simulink model "ORC_test_simu_unregSCIG"  (R2018a)
settings: Solver=FixedStepAuto  StartTime=0.0  StopTime=10  FixedStep=.1  RelTol=1e-4
values from neighbouring files (symbols this model uses):
  A_cond = 50    [Chena_ORC_test_simu_init.m]    (also in ORC_test_simu_init.m = 18.6)
  A_evap = 30    [Chena_ORC_test_simu_init.m]    (also in ORC_test_simu_init.m = 9.3)
  Cx = 620e-05    (= 0.0062)    [Chena_ORC_test_simu_init.m]    (also in ORC_test_simu_init.m = 0.000221048532072; SCIG_Admittance_Balance.m = 6.9e-05; SCIG_Energy_Balance_excitation.m = 1.35135135135; SCIG_Energy_Balance_excitation_sym.m = 5)
  eff_inverter = 0.93    [Chena_ORC_test_simu_init.m]    (also in ORC_test_simu_init.m)
  eff_pump = 0.78    [Chena_ORC_test_simu_init.m]    (also in ORC_Energy_Balance.m = 0.7; ORC_test.m = 0.7; ORC_test_brownfield.m = 0.7; ORC_test_greenfield.m = 0.7)
  eff_turbine = 0.8    [Chena_ORC_test_simu_init.m]    (also in ORC_test_simu_init.m = 0.78)
  f_rated = 60    [Chena_ORC_test_simu_init.m]    (also in ORC_test_simu_init.m; SCIG_Admittance_Balance.m; SCIG_Admittance_test.m; SCIG_Ouazenne.m)
  H_wf_init = 2.6e+05    (= 260000)    [Chena_ORC_test_simu_init.m]    (also in ORC_test_simu_init.m = 230000)
  Lr = 0.252/(2*pi*f_rated)/35    (= 1.9098593171e-05)    [Chena_ORC_test_simu_init.m]    (also in ORC_test_simu_init.m = 0.000132629119243)
  Ls = 0.423/(2*pi*f_rated)/35    (= 3.20583528228e-05)    [Chena_ORC_test_simu_init.m]    (also in ORC_test_simu_init.m = 0.000848826363157)
  m_dot_source = 33.39    [Chena_ORC_test_simu_init.m]    (also in ORC_Energy_Balance.m = 5.7714; ORC_test.m = 12; ORC_test_brownfield.m = 6; ORC_test_greenfield.m = 12)
  m_dot_wf_init = 12    [Chena_ORC_test_simu_init.m]    (also in ORC_test_simu_init.m = 3)
  m_dot_wf_max = 16    [Chena_ORC_test_simu_init.m]
  magCurveV = [98.1532063054068,98.8036071709152,99.4518999785459,100.098037520928,100.741973127402,101.383660677656,102.023054614968,102.660109959042,103.294782318460,103.927027902737,104.556803533993,105.184066658235,105.808775356268,106.430888354220,107.050365033694,107.667165441552,108.281250299330,108.892581012284,109.501119678081,110.106829095126,110.709672770539,111.309614927775,111.906620513896,112.5006 ...(+6146 chars)    [Chena_ORC_test_simu_init.m]    (also in ORC_test_simu_init.m = [21.5410077151772,22.1687511430959,22.7961934111159,23.42344)
  magCurveX = [0.663529769645709,0.663521969965503,0.663500208426959,0.663464444749194,0.663414643227627,0.663350772676200,0.663272806369214,0.663180721982808,0.663074501536138,0.662954131332260,0.662819601898778,0.662670907928276,0.662508048218555,0.662331025612717,0.662139846939116,0.661934522951205,0.661715068267290,0.661481501310239,0.661233844247137,0.660972122928937,0.660696366830103,0.660406608988283,0.6 ...(+6531 chars)    [Chena_ORC_test_simu_init.m]    (also in ORC_test_simu_init.m = [21.5410077151772,21.5637559851946,21.5850104594817,21.60498)
  p_atm = 101325    [Chena_ORC_test_simu_init.m]    (also in ORC_test_simu_init.m)
  pf_grid = 0.9    [Chena_ORC_test_simu_init.m]    (also in ORC_test_simu_init.m)
  poles = 2    [Chena_ORC_test_simu_init.m]    (also in Copy_of_SCIG_Energy_Balance_excitation.m = 4; SCIG_Admittance_Balance.m = 6; SCIG_Admittance_test.m = 6; SCIG_Ouazenne.m)
  Rr = 0.144/35    (= 0.00411428571429)    [Chena_ORC_test_simu_init.m]    (also in ORC_test_simu_init.m = 0.03)
  Rs = 0.148/35    (= 0.00422857142857)    [Chena_ORC_test_simu_init.m]    (also in ORC_test_simu_init.m = 0.018)
  Rx = 0    [Chena_ORC_test_simu_init.m]    (also in Copy_of_SCIG_Energy_Balance_excitation.m = 0.003; ORC_test_simu_init.m; SCIG_Admittance_Balance.m; SCIG_Admittance_test.m)
  Tin_sink = 277.59    [Chena_ORC_test_simu_init.m]    (also in ORC_test_simu_init.m = 278)
  Tin_source = 346.48    [Chena_ORC_test_simu_init.m]    (also in ORC_test_simu_init.m = 368)
  U_cond = 5000    [Chena_ORC_test_simu_init.m]    (also in ORC_test_simu_init.m = 1400)
  U_evap = 4500    [Chena_ORC_test_simu_init.m]    (also in ORC_test_simu_init.m = 1500)
  Vline_rated = 220    [Chena_ORC_test_simu_init.m]    (also in SCIG_Admittance_Balance.m = 6600; SCIG_Admittance_test.m = 6600; SCIG_Ouazenne.m; SCIG_Ouazenne_iterate.m)
  Xx = 1/(2*pi*f_rated*Cx)    (= 0.427835868527)    [Chena_ORC_test_simu_init.m]    (also in Copy_of_SCIG_Energy_Balance_excitation.m = 12; ORC_test_simu_init.m = 12; SCIG_Admittance_Balance.m = Xx(fvIDX); SCIG_Energy_Balance_excitation.m = 1./(Cx.*w_synch))
undefined symbols (not defined in the file or in its folder): handle_sink, handle_source, handle_wf, n_mech_init, n_mech_max, n_mech_min, sigbuilder_block
(part 1 of 4)
settings Model: Creator=njgreen3  LastModifiedBy=njgreen3
settings SolverCC: AlgebraicLoopSolver=LineSearch
settings DebuggingCC: ParameterOverflowMsg=warning

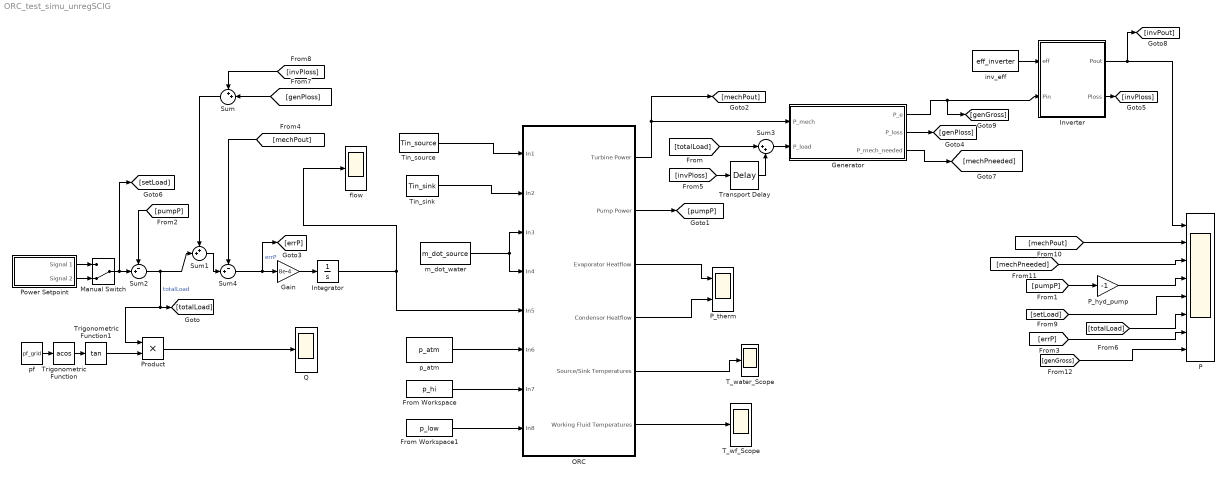
== system ORC_test_simu_unregSCIG ==
  From Workspace : FromWorkspace  VariableName=p_hi  SampleTime=0
  From Workspace1 : FromWorkspace  VariableName=p_low  SampleTime=0
  Gain : Gain  Gain=8e-4
  Generator : Subsystem
  Integrator : Integrator  InitialCondition=m_dot_wf_init  LimitOutput=on  UpperSaturationLimit=m_dot_wf_max  LowerSaturationLimit=0
  Inverter : MATLAB Function  TreatAsAtomicUnit=on
  Manual Switch : ManualSwitch  CurrentSetting=0
  ORC : Subsystem
  P : Scope  NumInputPorts=8
  P_hyd_pump : Gain  Gain=-1
  P_therm : Scope  NumInputPorts=2
  Power Setpoint : Subsystem  Tag=STV Subsys  LoadFcn=sigbuilder_block('load',[440.25 156.75 544.5 355.5 ]);  StartFcn=sigbuilder_block('start');  StopFcn=sigbuilder_block('stop');  ClipboardFcn=sigbuilder_block('clipboard');  mask(Sigbuilder block){tuvar=[0:10]}
      mask help: Simulink:masks:SigbuilderBlock_MD
      mask init:
      | if ~strcmp(get_param(bdroot(gcbh),'SimulationStatus'),'stopped') tuvar = sigbuilder_block('maskInit'); end
      settings: CopyFcn=sigbuilder_block('copy');  DeleteFcn=sigbuilder_block('delete');  ModelCloseFcn=sigbuilder_block('modelClose');  PreSaveFcn=sigbuilder_block('preSave');  PauseFcn=sigbuilder_block('pause');  ContinueFcn=sigbuilder_block('continue');  NameChangeFcn=sigbuilder_block('namechange');  OpenFcn=sigbuilder_block('open',[440.25 156.75 544.5 355.5 ]);  CloseFcn=sigbuilder_block('close');
      mask Display: plot(0, 0, 100, 100,[2, 2, 32, 32, 2], [68, 8, 8, 68, 68],[32, 2], [38, 38], [32, 19, 2],[53, 60, 44], [32, 17, 17, 2],[16, 16, 31, 31]);txt = getActiveGroup(gcbh);text(2, 100, txt,'verticalAlignment', 'top');
  Product : Product
  Q : Scope
  Sum : Sum  Inputs=++|
  Sum1 : Sum  Inputs=++|
  Sum2 : Sum  Inputs=-+|
  Sum3 : Sum  Inputs=|++
  Sum4 : Sum  Inputs=-+|
  T_water_Scope : Scope
  T_wf_Scope : Scope
  Tin_sink : Constant  Value=Tin_sink
  Tin_source : Constant  Value=Tin_source
  Transport Delay : TransportDelay  DelayTime=.01
  Trigonometric Function : Trigonometry  Operator=acos
  Trigonometric Function1 : Trigonometry  Operator=tan
  flow : Scope
  inv_eff : Constant  Value=eff_inverter
  m_dot_water : Constant  Value=m_dot_source
  p_atm : Constant  Value=p_atm
  pf : Constant  Value=pf_grid
  wires:
  Tin_source/1 -> ORC/1(In1)
  m_dot_water/1 -> ORC/3(In3), ORC/4(In4)
  p_atm/1 -> ORC/6(In6)
  From Workspace/1 -> ORC/7(In7)
  From Workspace1/1 -> ORC/8(In8)
  ORC/3(Evaporator Heatflow) -> P_therm/1
  ORC/4(Condensor Heatflow) -> P_therm/2
  ORC/5(Source/Sink Temperatures) -> T_water_Scope/1
  ORC/6(Working Fluid Temperatures) -> T_wf_Scope/1
  Tin_sink/1 -> ORC/2(In2)
  Gain/1 -> Integrator/1
  Power Setpoint/1(Signal 1) -> Manual Switch/1
  Power Setpoint/2(Signal 2) -> Manual Switch/2
  Manual Switch/1 -> [setLoad], Sum2/2
  pf/1 -> Trigonometric Function/1
  Trigonometric Function/1 -> Trigonometric Function1/1
  Trigonometric Function1/1 -> Product/2
  Product/1 -> Q/1
  Sum2/1 -> Sum1/2, Product/1, [totalLoad]  "totalLoad"
  Integrator/1 -> ORC/5(In5), flow/1
  P_hyd_pump/1 -> P/4
  Sum4/1 -> [errP], Gain/1  "errP"
  inv_eff/1 -> Inverter/1(eff)
  Generator/2(P_loss) -> [genPloss]
  Generator/1(P_e) -> [genGross], Inverter/2(Pin)
  Generator/3(P_mech_needed) -> [mechPneeded]
  Sum/1 -> Sum1/1
  [totalLoad] -> Sum3/1
  ORC/2(Pump Power) -> [pumpP]
  [pumpP] -> P_hyd_pump/1
  [pumpP] -> Sum2/1
  [errP] -> P/7
  [mechPout] -> Sum4/1
  [totalLoad] -> P/6
  [genPloss] -> Sum/2
  Inverter/2(Ploss) -> [invPloss]
  [invPloss] -> Sum/1
  [setLoad] -> P/5
  [mechPout] -> P/2
  Inverter/1(Pout) -> [invPout], P/1
  ORC/1(Turbine Power) -> [mechPout], Generator/1(P_mech)
  [mechPneeded] -> P/3
  Sum1/1 -> Sum4/2
  Transport Delay/1 -> Sum3/2
  Sum3/1 -> Generator/2(P_load)
  [invPloss] -> Transport Delay/1
  [genGross] -> P/8

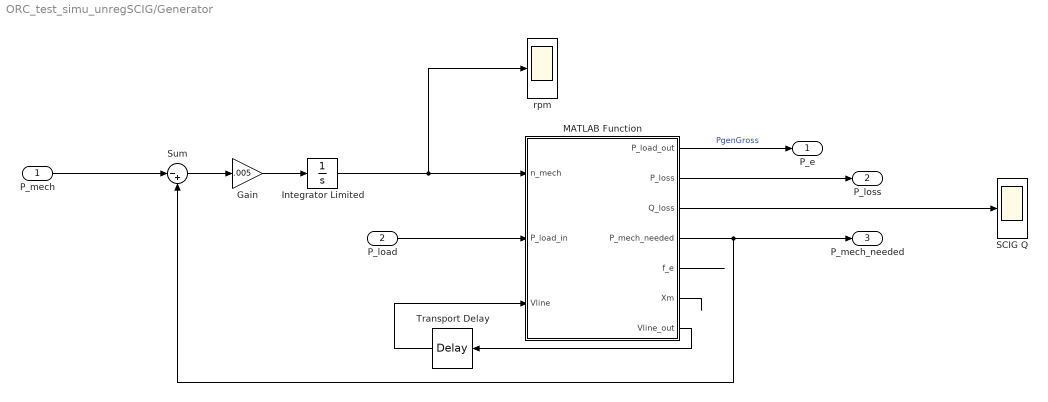
== system ORC_test_simu_unregSCIG/Generator ==
  P_mech : Inport
  P_load : Inport  Port=2
  Gain : Gain  Gain=.005
  Integrator Limited : Integrator  InitialCondition=n_mech_init  LimitOutput=on  UpperSaturationLimit=n_mech_max  LowerSaturationLimit=n_mech_min
  MATLAB Function : MATLAB Function  mask{Vline_rated=Vline_rated, f_rated=f_rated, poles=poles, R1=Rs, L1=Ls, R2=Rr, L2=Lr, magCurveX=magCurveX, magCurveV=magCurveV, Rx=Rx, Xx=Xx, K_b=0, K_w=0}
      mask prompts: Vline_rated "Line Voltage (V)"; f_rated "Frequency (Hz)"; R1 "Stator Resistance, Rs"; L1 "Stator Inductance, Ls"; R2 "Referred Rotor Resistance, Rr'"; L2 "Referred Rotor Inductance, Lr'"; magCurveX "Magnetization Reactance Curve, Xm"; magCurveV "Magnetizing Voltage Curve, Vg"; Rx "Equivalent Series Resistance (ESR) of excitationm, Rx"; Xx "Excitation capacitance, Xx"; K_b "Coefficient of Bearing Friction, Kb"; K_w "Coefficient of Windage Friction, Kw"
  SCIG Q : Scope
  Sum : Sum  Inputs=|-+
  Transport Delay : TransportDelay  DelayTime=.01  InitialOutput=Vline_rated
  rpm : Scope
  P_e : Outport
  P_loss : Outport  Port=2
  P_mech_needed : Outport  Port=3
  wires:
  Integrator Limited/1 -> MATLAB Function/1(n_mech), rpm/1
  Transport Delay/1 -> MATLAB Function/3(Vline)
  P_mech/1 -> Sum/1
  MATLAB Function/1(P_load_out) -> P_e/1  "PgenGross"
  MATLAB Function/2(P_loss) -> P_loss/1
  MATLAB Function/7(Vline_out) -> Transport Delay/1
  P_load/1 -> MATLAB Function/2(P_load_in)
  MATLAB Function/3(Q_loss) -> SCIG Q/1
  MATLAB Function/4(P_mech_needed) -> Sum/2, P_mech_needed/1
  MATLAB Function/6(Xm) -> ?
  MATLAB Function/5(f_e) -> ?
  Sum/1 -> Gain/1
  Gain/1 -> Integrator Limited/1

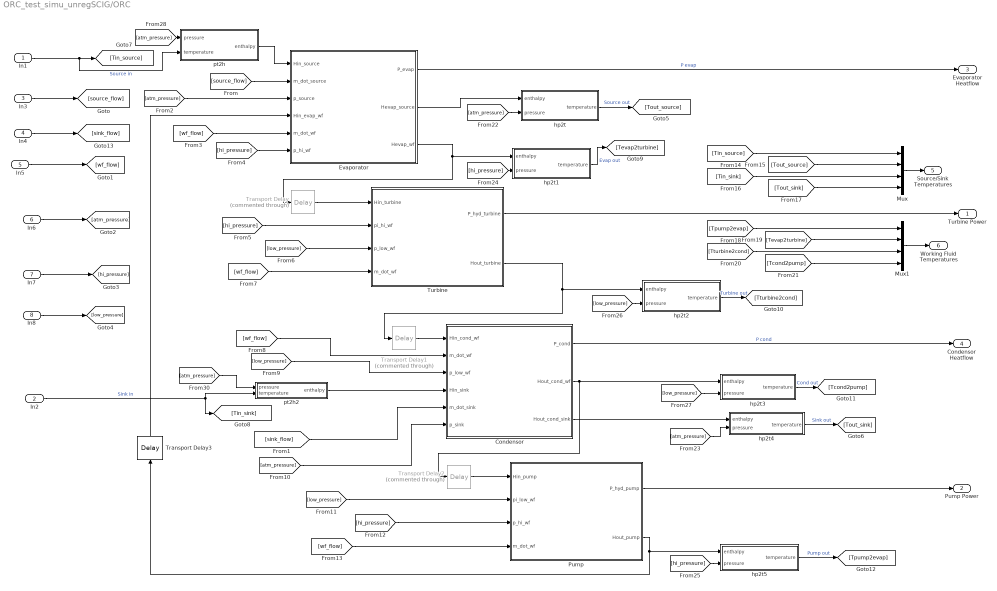
== system ORC_test_simu_unregSCIG/ORC ==
  In1 : Inport
  In2 : Inport  Port=2
  In3 : Inport  Port=3
  In4 : Inport  Port=4
  In5 : Inport  Port=5
  In6 : Inport  Port=6
  In7 : Inport  Port=7
  In8 : Inport  Port=8
  Condensor : Subsystem
  Evaporator : Subsystem
  Mux : Mux
  Mux1 : Mux
  Pump : Subsystem
  Transport Delay : TransportDelay  Commented=through  DelayTime=.01  InitialOutput=2.3e+05
  Transport Delay1 : TransportDelay  Commented=through  DelayTime=.01  InitialOutput=2.3e+05
  Transport Delay2 : TransportDelay  Commented=through  DelayTime=.01  InitialOutput=2.3e+05
  Transport Delay3 : TransportDelay  DelayTime=.01  InitialOutput=H_wf_init  TransDelayFeedthrough=on
  Turbine : Subsystem
  hp2t : MATLAB Function  TreatAsAtomicUnit=on  mask{fluid_handle=handle_source}
      mask prompts: fluid_handle "Fluid Handle"
  hp2t1 : MATLAB Function  TreatAsAtomicUnit=on  mask{fluid_handle=handle_wf}
      mask prompts: fluid_handle "Fluid Handle"
  hp2t2 : MATLAB Function  TreatAsAtomicUnit=on  mask{fluid_handle=handle_wf}
      mask prompts: fluid_handle "Fluid Handle"
  hp2t3 : MATLAB Function  TreatAsAtomicUnit=on  mask{fluid_handle=handle_wf}
      mask prompts: fluid_handle "Fluid Handle"
  hp2t4 : MATLAB Function  TreatAsAtomicUnit=on  mask{fluid_handle=handle_sink}
      mask prompts: fluid_handle "Fluid Handle"
  hp2t5 : MATLAB Function  TreatAsAtomicUnit=on  mask{fluid_handle=handle_wf}
      mask prompts: fluid_handle "Fluid Handle"
  pt2h : MATLAB Function  TreatAsAtomicUnit=on  mask{fluid_handle=handle_source}
      mask prompts: fluid_handle "Fluid Handle"
  pt2h2 : MATLAB Function  TreatAsAtomicUnit=on  mask{fluid_handle=handle_sink}
      mask prompts: fluid_handle "Fluid Handle"
  Turbine Power : Outport
  Pump Power : Outport  Port=2
  Evaporator Heatflow : Outport  Port=3
  Condensor Heatflow : Outport  Port=4
  Source/Sink Temperatures : Outport  Port=5
  Working Fluid Temperatures : Outport  Port=6
  wires:
  [wf_flow] -> Pump/4(m_dot_wf)
  Pump/2(Hout_pump) -> Transport Delay3/1, hp2t5/1(enthalpy)
  [Tturbine2cond] -> Mux1/3
  Condensor/2(Hout_cond_wf) -> hp2t3/1(enthalpy), Transport Delay2/1
  Transport Delay1/1 -> Condensor/1(Hin_cond_wf)
  In3/1 -> [source_flow]
  Transport Delay3/1 -> Evaporator/4(Hin_evap_wf)
  [atm_pressure] -> Evaporator/3(p_source)
  Evaporator/3(Hevap_wf) -> Transport Delay/1, hp2t1/1(enthalpy)
  Transport Delay/1 -> Turbine/1(Hin_turbine)
  In1/1 -> pt2h/2(temperature), [Tin_source]  "Source in"
  hp2t2/1(temperature) -> [Tturbine2cond]  "Turbine out"
  [atm_pressure] -> hp2t4/2(pressure)
  [wf_flow] -> Evaporator/5(m_dot_wf)
  [hi_pressure] -> Pump/3(p_hi_wf)
  Turbine/2(Hout_turbine) -> Transport Delay1/1, hp2t2/1(enthalpy)
  [low_pressure] -> Condensor/3(p_low_wf)
  [hi_pressure] -> Evaporator/6(p_hi_wf)
  [low_pressure] -> Turbine/3(p_low_wf)
  [wf_flow] -> Turbine/4(m_dot_wf)
  [wf_flow] -> Condensor/2(m_dot_wf)
  [Tcond2pump] -> Mux1/4
  [sink_flow] -> Condensor/5(m_dot_sink)
  [atm_pressure] -> Condensor/6(p_sink)
  Evaporator/2(Hevap_source) -> hp2t/1(enthalpy)
  [low_pressure] -> hp2t3/2(pressure)
  [hi_pressure] -> Turbine/2(pi_hi_wf)
  [atm_pressure] -> pt2h/1(pressure)
  Transport Delay2/1 -> Pump/1(Hin_pump)
  hp2t4/1(temperature) -> [Tout_sink]  "Sink out"
  hp2t/1(temperature) -> [Tout_source]  "Source out"
  [low_pressure] -> Pump/2(pi_low_wf)
  hp2t1/1(temperature) -> [Tevap2turbine]  "Evap out"
  hp2t3/1(temperature) -> [Tcond2pump]  "Cond out"
  hp2t5/1(temperature) -> [Tpump2evap]  "Pump out"
  [low_pressure] -> hp2t2/2(pressure)
  [hi_pressure] -> hp2t5/2(pressure)
  [source_flow] -> Evaporator/2(m_dot_source)
  [atm_pressure] -> pt2h2/1(pressure)
  [hi_pressure] -> hp2t1/2(pressure)
  [atm_pressure] -> hp2t/2(pressure)
  pt2h2/1(enthalpy) -> Condensor/4(Hin_sink)
  Condensor/3(Hout_cond_sink) -> hp2t4/1(enthalpy)
  pt2h/1(enthalpy) -> Evaporator/1(Hin_source)
  In2/1 -> pt2h2/2(temperature), [Tin_sink]  "Sink in"
  [Tout_source] -> Mux/2
  In7/1 -> [hi_pressure]
  In5/1 -> [wf_flow]
  In8/1 -> [low_pressure]
  In6/1 -> [atm_pressure]
  [Tin_source] -> Mux/1
  [Tin_sink] -> Mux/3
  [Tevap2turbine] -> Mux1/2
  Evaporator/1(P_evap) -> Evaporator Heatflow/1  "P evap"
  Pump/1(P_hyd_pump) -> Pump Power/1
  Condensor/1(P_cond) -> Condensor Heatflow/1  "P cond"
  [Tpump2evap] -> Mux1/1
  Turbine/1(P_hyd_turbine) -> Turbine Power/1
  [Tout_sink] -> Mux/4
  Mux/1 -> Source/Sink Temperatures/1
  Mux1/1 -> Working Fluid Temperatures/1
  In4/1 -> [sink_flow]

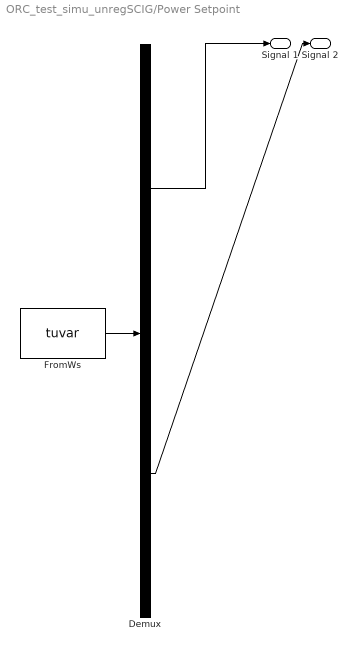
== system ORC_test_simu_unregSCIG/Power Setpoint ==
  Demux : Demux  Tag=STV Demux  Outputs=2
  FromWs : FromWorkspace  Tag=STV FromWs  VariableName=tuvar  SampleTime=0
      SigBuilderData=|
      | common.afterFinalStr = 'Extrapolate'
      | common.sampleTime = 0
      | dataSet.timeRange = [0 62]
      | dataSet.name = 'Group 1'
      | sbobj.Groups.Name = 'Group 1'
      | sbobj.Groups.Signals(1).Name = 'Signal 1'
      | sbobj.Groups.Signals(1).XData = [0 2 2 4 4 6 6 8 8 10 10 62]
      | sbobj.Groups.Signals(1).YData = [20000 20000 22000 22000 24000 24000 26000 26000 28000 27900 27800 15500]
      | sbobj.Groups.Signals(2).Name = 'Signal 2'
      | sbobj.Groups.Signals(2).XData = [0 62]
      | sbobj.Groups.Signals(2).YData = [35000 35000]
      | sbobj.Groups.TimeRange = [0 62]
  Signal 1 : Outport  Tag=STV Outport
  Signal 2 : Outport  Tag=STV Outport  Port=2
  wires:
  Demux/1 -> Signal 1/1
  FromWs/1 -> Demux/1
  Demux/2 -> Signal 2/1

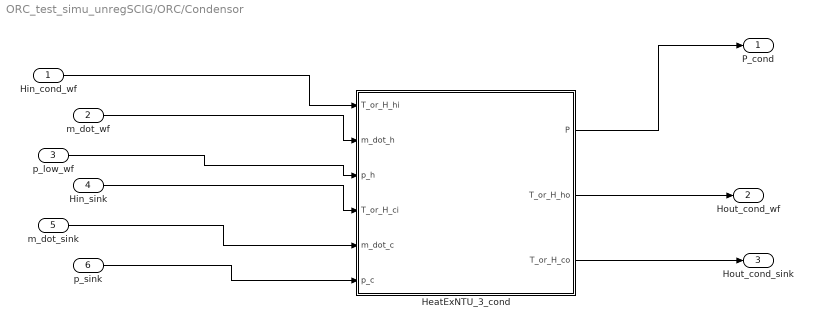
== system ORC_test_simu_unregSCIG/ORC/Condensor ==
  Hin_cond_wf : Inport
  m_dot_wf : Inport  Port=2
  p_low_wf : Inport  Port=3
  Hin_sink : Inport  Port=4
  m_dot_sink : Inport  Port=5
  p_sink : Inport  Port=6
  HeatExNTU_3_cond : MATLAB Function  Description=|  TreatAsAtomicUnit=on  mask{U=U_cond, A=A_cond, HeatExType=counter, fluid_h=handle_wf, fluid_c=handle_sink, T_or_H=0}
      | %HeatExNTU Summary 
      | %   This function calculates flow and outlet temperatures of a heat exchanger
      | %   using the Number of Transfer Units (NTU) method as described in
      | %   Fundementals of Heat and Mass Transfer by F. P. Incropera, D. P.
      | %   DeWitt, T. L. Bergman & A. S. Lavine. The method can be used when only
      | %   the inlet tempertures are known as opposed to inlet and outlet
      | %   temperatures.
      | %
      | %   This is done by calculating effectiveness which is defined as the ratio
      | %   of actual heat transferred to the maximum possible heat transferred for 
      | %   an infinite length counter-flow heat exchanger with the given inlet
      | %   temperatures. The effectivenes is calculated differently depending on 
      | %   the geometry of exchanger but is always a function of the ratio of heat
      | %   capacity rates as well as the number of transfer units (NTU). The NTU
      | %   depends on the overall heat transfer coefficient, the heat transfer
      | %   area, and the smaller of the two heat capacity rates. 
      | %   
      | %   In the event of a phase change the rate of change of energy required to
      | %   get the fluid just beyond the point of vaporizaion or condensation is
      | %   calculated using the CoolProp function. Then the function is called
      | %   again at the new temperature and the final temperatures and heat rates
      | %   are calucluated using a reduced heat exhange area. I currently assume
      | %   the effected heat transfer area is a half of the original input. This 
      | %   function cannot accurately handle both fluids changing phase because it
      | %   does not check which fluid would change first.
      | % 
      | % Note: The effectiveness is separte from efficiency. The calculations
      | %   assumes an efficiency of 1 where all heat is transferred from the hot
      | %   fluid to the cool fluid or remains within the the fluid. This also
      | %   assumes no fluid is undergoing a change in state, which may not be
      | %   sufficient for my final model.
      | %
      | % This function makes use of the CoolProp wrapper for fluid properties. 
      | % The high level Matlab wrapper cannot handle vector inputs. There ways to
      | % make low level calls interfacing with the DLL so many values can be
      | % determined more quickly, but that is not implented here.
      | % More information about the Matlab wrapper can be found at
      | %   http://www.coolprop.org/coolprop/wrappers/MATLAB/index.html
      | % A list of parameters can be found at 
      | %   http://www.coolprop.org/coolprop/HighLevelAPI.html#parameter-table
      | % A list of fluids can be found at 
      | %   http://www.coolprop.org/fluid_properties/PurePseudoPure.html#list-of-fluids
      | %
      | % Inputs:
      | %   Thi         Hot fluid inlet temperature in Kelvin
      | %   m_dot_h     Hot fluid mass flow rate in kg/s
      | %   p_h         Hot fluid pressure in pa
      | %   fluid_h     Name of Hot fluid (string)
      | %   Tci         Cool fluid inlet temperature in Kelvin
      | %   m_dot_c     Cool fluid mass flow rate in kg/s
      | %   p_c         Cool fluid pressure in pa
      | %   fluid_c     Name of Cool fluid (string)
      | %   HeatExType  String describing the heat exchanger geometry. Currently
      | %               this variable only accepts 'counter' and 'parallel', but
      | %               can be expanded to other exchanger/flow types
      | %               'counter' for counter flow
      | %               'parallel' for parallel
      | %   U           Overall heat transfer coefficient in W/(K m2)
      | %   A           Heat transfer area in m2
      | %
      | % Output:
      | %   P           Rate of heat exchenged (power) in W
      | %   Tho         Hot fluid outlet temperature in input temp units (K)
      | %   Tco         Cool fluid outlet temperature in input tempt units (K)
      mask prompts: U "Heat Transfer Coefficient"; A "Heat Transfer Area"; HeatExType "Heat Exchanger Type"; fluid_h "Hot Fluid Handle"; fluid_c "Cool Fluid Handle"; T_or_H "Temperature(1) or Enthalpy(0)"
  P_cond : Outport
  Hout_cond_wf : Outport  Port=2
  Hout_cond_sink : Outport  Port=3
  wires:
  Hin_cond_wf/1 -> HeatExNTU_3_cond/1(T_or_H_hi)
  m_dot_wf/1 -> HeatExNTU_3_cond/2(m_dot_h)
  p_low_wf/1 -> HeatExNTU_3_cond/3(p_h)
  p_sink/1 -> HeatExNTU_3_cond/6(p_c)
  m_dot_sink/1 -> HeatExNTU_3_cond/5(m_dot_c)
  Hin_sink/1 -> HeatExNTU_3_cond/4(T_or_H_ci)
  HeatExNTU_3_cond/1(P) -> P_cond/1
  HeatExNTU_3_cond/2(T_or_H_ho) -> Hout_cond_wf/1
  HeatExNTU_3_cond/3(T_or_H_co) -> Hout_cond_sink/1

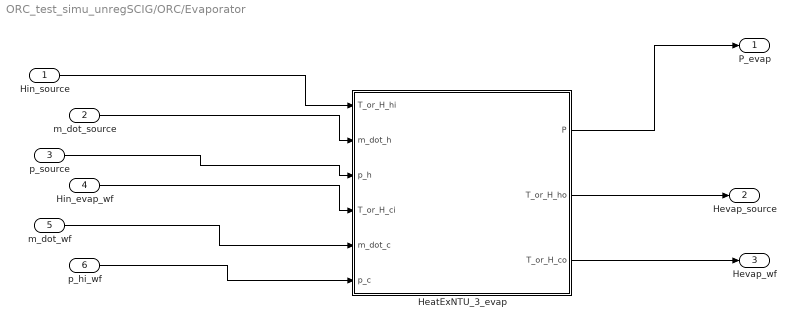
== system ORC_test_simu_unregSCIG/ORC/Evaporator ==
  Hin_source : Inport
  m_dot_source : Inport  Port=2
  p_source : Inport  Port=3
  Hin_evap_wf : Inport  Port=4
  m_dot_wf : Inport  Port=5
  p_hi_wf : Inport  Port=6
  HeatExNTU_3_evap : MATLAB Function  Description=|  TreatAsAtomicUnit=on  mask{U=U_evap, A=A_evap, HeatExType=counter, fluid_h=handle_source, fluid_c=handle_wf, T_or_H=0}
      | %HeatExNTU Summary 
      | %   This function calculates flow and outlet temperatures of a heat exchanger
      | %   using the Number of Transfer Units (NTU) method as described in
      | %   Fundementals of Heat and Mass Transfer by F. P. Incropera, D. P.
      | %   DeWitt, T. L. Bergman & A. S. Lavine. The method can be used when only
      | %   the inlet tempertures are known as opposed to inlet and outlet
      | %   temperatures.
      | %
      | %   This is done by calculating effectiveness which is defined as the ratio
      | %   of actual heat transferred to the maximum possible heat transferred for 
      | %   an infinite length counter-flow heat exchanger with the given inlet
      | %   temperatures. The effectivenes is calculated differently depending on 
      | %   the geometry of exchanger but is always a function of the ratio of heat
      | %   capacity rates as well as the number of transfer units (NTU). The NTU
      | %   depends on the overall heat transfer coefficient, the heat transfer
      | %   area, and the smaller of the two heat capacity rates. 
      | %   
      | %   In the event of a phase change the rate of change of energy required to
      | %   get the fluid just beyond the point of vaporizaion or condensation is
      | %   calculated using the CoolProp function. Then the function is called
      | %   again at the new temperature and the final temperatures and heat rates
      | %   are calucluated using a reduced heat exhange area. I currently assume
      | %   the effected heat transfer area is a half of the original input. This 
      | %   function cannot accurately handle both fluids changing phase because it
      | %   does not check which fluid would change first.
      | % 
      | % Note: The effectiveness is separte from efficiency. The calculations
      | %   assumes an efficiency of 1 where all heat is transferred from the hot
      | %   fluid to the cool fluid or remains within the the fluid. This also
      | %   assumes no fluid is undergoing a change in state, which may not be
      | %   sufficient for my final model.
      | %
      | % This function makes use of the CoolProp wrapper for fluid properties. 
      | % The high level Matlab wrapper cannot handle vector inputs. There ways to
      | % make low level calls interfacing with the DLL so many values can be
      | % determined more quickly, but that is not implented here.
      | % More information about the Matlab wrapper can be found at
      | %   http://www.coolprop.org/coolprop/wrappers/MATLAB/index.html
      | % A list of parameters can be found at 
      | %   http://www.coolprop.org/coolprop/HighLevelAPI.html#parameter-table
      | % A list of fluids can be found at 
      | %   http://www.coolprop.org/fluid_properties/PurePseudoPure.html#list-of-fluids
      | %
      | % Inputs:
      | %   Thi         Hot fluid inlet temperature in Kelvin
      | %   m_dot_h     Hot fluid mass flow rate in kg/s
      | %   p_h         Hot fluid pressure in pa
      | %   fluid_h     Name of Hot fluid (string)
      | %   Tci         Cool fluid inlet temperature in Kelvin
      | %   m_dot_c     Cool fluid mass flow rate in kg/s
      | %   p_c         Cool fluid pressure in pa
      | %   fluid_c     Name of Cool fluid (string)
      | %   HeatExType  String describing the heat exchanger geometry. Currently
      | %               this variable only accepts 'counter' and 'parallel', but
      | %               can be expanded to other exchanger/flow types
      | %               'counter' for counter flow
      | %               'parallel' for parallel
      | %   U           Overall heat transfer coefficient in W/(K m2)
      | %   A           Heat transfer area in m2
      | %
      | % Output:
      | %   P           Rate of heat exchenged (power) in W
      | %   Tho         Hot fluid outlet temperature in input temp units (K)
      | %   Tco         Cool fluid outlet temperature in input tempt units (K)
      mask prompts: U "Heat Transfer Coefficient"; A "Heat Transfer Area"; HeatExType "Heat Exchanger Type"; fluid_h "Hot Fluid Handle"; fluid_c "Cool Fluid Handle"; T_or_H "Temperature (1) or Enthalpy (0)"
      mask init:
      | % set_param('ORC_test_simu/Evaporator/HeatExNTU_3_block', 'fluid_h', 'Water')
  P_evap : Outport
  Hevap_source : Outport  Port=2
  Hevap_wf : Outport  Port=3
  wires:
  Hin_source/1 -> HeatExNTU_3_evap/1(T_or_H_hi)
  m_dot_source/1 -> HeatExNTU_3_evap/2(m_dot_h)
  p_source/1 -> HeatExNTU_3_evap/3(p_h)
  p_hi_wf/1 -> HeatExNTU_3_evap/6(p_c)
  m_dot_wf/1 -> HeatExNTU_3_evap/5(m_dot_c)
  Hin_evap_wf/1 -> HeatExNTU_3_evap/4(T_or_H_ci)
  HeatExNTU_3_evap/1(P) -> P_evap/1
  HeatExNTU_3_evap/2(T_or_H_ho) -> Hevap_source/1
  HeatExNTU_3_evap/3(T_or_H_co) -> Hevap_wf/1

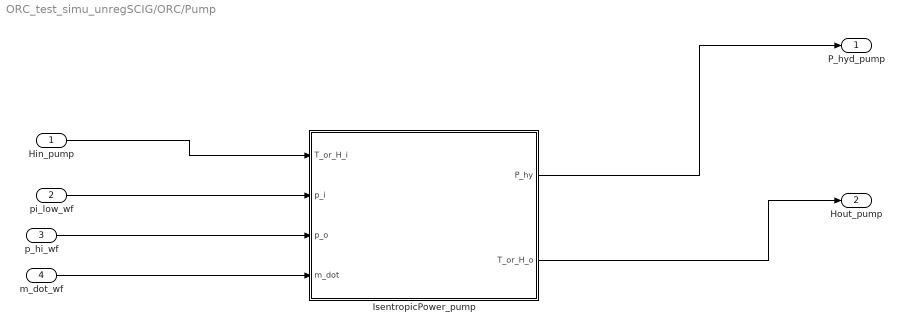
== system ORC_test_simu_unregSCIG/ORC/Pump ==
  Hin_pump : Inport
  pi_low_wf : Inport  Port=2
  p_hi_wf : Inport  Port=3
  m_dot_wf : Inport  Port=4
  IsentropicPower_pump : MATLAB Function  TreatAsAtomicUnit=on  mask{isen_eff=eff_pump, T_or_H=0, fluid=handle_wf}
      mask prompts: isen_eff "Isentropic Efficiency"; T_or_H "Temperature (1) or Enthalpy (0)"; fluid "Fluid Handle"
  P_hyd_pump : Outport
  Hout_pump : Outport  Port=2
  wires:
  pi_low_wf/1 -> IsentropicPower_pump/2(p_i)
  m_dot_wf/1 -> IsentropicPower_pump/4(m_dot)
  Hin_pump/1 -> IsentropicPower_pump/1(T_or_H_i)
  IsentropicPower_pump/1(P_hy) -> P_hyd_pump/1
  IsentropicPower_pump/2(T_or_H_o) -> Hout_pump/1
  p_hi_wf/1 -> IsentropicPower_pump/3(p_o)

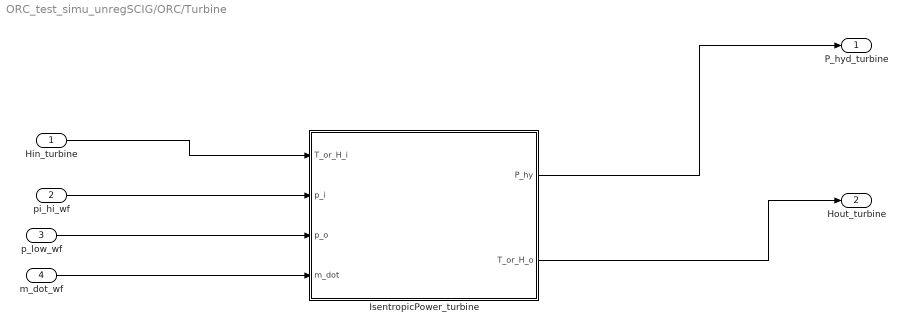
== system ORC_test_simu_unregSCIG/ORC/Turbine ==
  Hin_turbine : Inport
  pi_hi_wf : Inport  Port=2
  p_low_wf : Inport  Port=3
  m_dot_wf : Inport  Port=4
  IsentropicPower_turbine : MATLAB Function  TreatAsAtomicUnit=on  mask{isen_eff=eff_turbine, T_or_H=0, fluid=handle_wf}
      mask prompts: isen_eff "Isentropic Efficiency"; T_or_H "Temperature (1) or Enthalpy (0)"; fluid "Fluid Handle"
  P_hyd_turbine : Outport
  Hout_turbine : Outport  Port=2
  wires:
  pi_hi_wf/1 -> IsentropicPower_turbine/2(p_i)
  m_dot_wf/1 -> IsentropicPower_turbine/4(m_dot)
  Hin_turbine/1 -> IsentropicPower_turbine/1(T_or_H_i)
  IsentropicPower_turbine/1(P_hy) -> P_hyd_turbine/1
  IsentropicPower_turbine/2(T_or_H_o) -> Hout_turbine/1
  p_low_wf/1 -> IsentropicPower_turbine/3(p_o)

== matlab function ORC_test_simu_unregSCIG/ORC/Turbine/IsentropicPower_turbine ==
  data: T_or_H_i input; P_hy output; p_i input; p_o input; m_dot input; T_or_H_o output; T_or_H parameter; isen_eff parameter; fluid parameter
function [ P_hy, T_or_H_o ] = IsentropicPower_block( T_or_H_i, p_i, p_o, m_dot, T_or_H,  isen_eff, fluid)
% function [ P_hy ] = IsentropicPower( T_i, T_o, p_i, p_o, m_dot, fluid, isen_eff )
%EXPANDER Summary of this function
%   This process calculates the mechanical power provided or required by a 
%   generic expander device/system. Turbines and other expanders provide
%   mechanical power while pumps and compressors consume it. This is done
%   by calculating the change in enthalpy of fluid and multipying by the 
%   mass flow rate while entropy remains constant.  Non ideal processes are
%   taken into account through the isentropic efficiency.
% 
% Inputs:
%   T_or_H_i    Input temperature in Kelvin or enthalpy in J/kg
%   p_i         Input pressure of the fluid in Pa
%   p_o         Output temperature of the fluid in Pa
%   m_dot       Mass flow rate of the fluid in kg/s 
%   fluid       Initialzed coolprop fluid handle
%   isen_eff    Isentropic efficiency of the device. Expected range: 0-1
%               This input is optional. If it is not provided then it will 
%               be set to 1, which is the efficiency of an ideal isentropic
%               device where entropy is constant.
%               This value is treated differently depending on if there is
%               an increase or decrease in fluid enthalpy. If the enthalpy
%               decreases (energy is extracted from the system) then the
%               efficiency if multiplied by the change in energy because
%               less energy is extracted than the ideal case. If the
%               enthalpy increases (energy in added to the system) then the
%               efficiency is divided by the change in energy because more
%               energy is required than the ideal case.
%   T_or_H      Logical indicating whether the relavent input and output
%               variables are temperature (1) or enthalpy (0)
% 
% Outputs:
%   P_hy        Hydraulic power exctracted or consumed in W. Positive
%               values indicate the system is providing hydraulic power as
%               a turbine or expander. Negative values indicate the system 
%               is consuming hydraulic power as a compressor or pump.
%   T_or_H_o    Output temperature in Kelvin or enthalpy in J/kg

% This function makes use of the CoolProp wrapper for fluid properties. 
% The high level Matlab wrapper cannot handle vector inputs. There ways to
% make low level calls interfacing with the DLL so many values can be
% determined more quickly, but that is not implented here.
% More information about the Matlab wrapper can be found at
%   http://www.coolprop.org/coolprop/wrappers/MATLAB/index.html
% A list of parameters can be found at 
%   http://www.coolprop.org/coolprop/HighLevelAPI.html#parameter-table
% A list of fluids can be found at 
%   http://www.coolprop.org/fluid_properties/PurePseudoPure.html#list-of-fluids

% initailize certain parameters used to call coolprop library
buffer_size = 255;
ierr = 0;
b = (1:1:buffer_size);
herr= char(b);
coder.extrinsic('calllib') 
coder.extrinsic('libpointer') 

% All the input signals should be the same size, so it shouldn't matter
% which one is used to obtain signal length
var_length = length(T_or_H_i);

% determine input parameter pair indecies for coolprop calls
% [pq_ind,~] = calllib('coolprop','get_input_pair_index','PQ_INPUTS'); %pressure and Mass vapor quality
[pt_ind,~] = calllib('coolprop','get_input_pair_index','PT_INPUTS'); %pressure and temperature
[hp_ind,~] = calllib('coolprop','get_input_pair_index','HmassP_INPUTS'); %Mass specific enthalpy and pressure
[ps_ind,~] = calllib('coolprop','get_input_pair_index','PSmass_INPUTS'); %pressure and Mass specific entropy

% determine output parameter indecies for coolprop calls
[t_ind, ~] = calllib('coolprop','get_param_index','T'); %temperature
[s_ind, ~] = calllib('coolprop','get_param_index','S'); %Mass specific entropy
[h_ind, ~] = calllib('coolprop','get_param_index','Hmass'); %Mass specific enthalpy
% [c_ind, ~] = calllib('coolprop','get_param_index','Cpmass'); %Mass specific constant pressure specific heat

% find pointer location of pressure input and output values
p_i_Ptr = libpointer('doublePtr',p_i);
p_o_Ptr = libpointer('doublePtr',p_o);

% Ensure temperature/enthalpy input variables are delt with appropriately
if T_or_H 
% Assume given temperature values are not at vaporization/condensation.
% Initialize T and H inputs
    T_i = T_or_H_i;
    T_i_Ptr = libpointer('doublePtr',T_i);
    H_i = zeros(var_length,1); % initialized to 0 temporarily
    H_i_Ptr = libpointer('doublePtr',H_i);
% Update values located at Hhi and Hci pointer locations
    calllib('coolprop','AbstractState_update_and_1_out', fluid, pt_ind, p_i_Ptr, T_i_Ptr, var_length, h_ind, H_i_Ptr, ierr,herr,buffer_size);
% Set Hhi & Hci to values stored at pointer location
    H_i = get(H_i_Ptr,'Value');
    
else
% Enthalpy values can be in vaporization/condensation region  
% Initialize H values
    H_i = T_or_H_i;
    H_i_Ptr = libpointer('doublePtr',H_i);

end

% Input entropy in J/kg/K
% Initialize pointer locations for relevant variables
S_i_Ptr = libpointer('doublePtr', zeros(var_length,1)); 
% Update values at S_i pointer location
calllib('coolprop','AbstractState_update_and_1_out', fluid, hp_ind, H_i_Ptr, p_i_Ptr, var_length, s_ind, S_i_Ptr, ierr,herr,buffer_size);
% Set S_i to values stored at pointer location
% S_i = get(S_i_Ptr,'Value');

% Ideal Output entropy is equal to input entropy 
% Ideal Output enthalpy in J/kg and temperature
H_o_ideal = zeros(var_length,1);
H_o_ideal_Ptr = libpointer('doublePtr',H_o_ideal);
% Update values located at Hhi and Hci pointer locations
calllib('coolprop','AbstractState_update_and_1_out', fluid, ps_ind, p_o_Ptr, S_i_Ptr, var_length, h_ind, H_o_ideal_Ptr, ierr,herr,buffer_size);
% Set H_o_ideal to values stored at pointer location
H_o_ideal = get(H_o_ideal_Ptr,'Value');

% Calculate Ideal power consumed/provided
P_ideal = m_dot.*(H_i - H_o_ideal);

% Initialize hydrolic power variable
P_hy = zeros(var_length,1);
%   If positive then the system is providing power as a turbine
%   or expander.
%   This means the actual power provided is less than the ideal power
P_hy(P_ideal > 0) = isen_eff.*P_ideal(P_ideal > 0);

%   If negative then the system is consuming power as a
%   compressor or pump.
%   This means the actual power consumed is greater than the ideal power.
P_hy(P_ideal < 0) = P_ideal(P_ideal < 0)./isen_eff;

% Set output enthalpy
H_o = H_i - P_hy./m_dot;
H_o_Ptr = libpointer('doublePtr',H_o);

% Ensure temperature/enthalpy input variables are delt with appropriately
if T_or_H 
% Assume given temperature values are not at vaporization/condensation
    T_or_H_o = zeros(var_length,1);
    T_or_H_o_Ptr = libpointer('doublePtr',T_or_H_o);
    calllib('coolprop','AbstractState_update_and_1_out', fluid, hp_ind, H_o_Ptr, p_o_Ptr, var_length, t_ind, T_or_H_o_Ptr, ierr,herr,buffer_size);
    T_or_H_o = get(T_or_H_o_Ptr,'Value');
    
else
% Enthalpy values can be in vaporization/condensation region    
    T_or_H_o = H_o;
end
end
